simulink model "Lightning_McSeas_VCU"  (R2021b)
settings: Solver=FixedStepDiscrete  StartTime=0.0  StopTime=10.0  FixedStep=0.01  RelTol=1e-3  EnableMultiTasking=on
PreLoadFcn:
  | try, model_open; catch, disp('Error occurred while executing model pre-load callback: model_open.m'); disp('Please assure that the MATLAB working directory is set to the model directory before opening.'); end
InitFcn:
  | try, model_open; catch, end
undefined symbols (not defined in the file): dataName, enumName, enumValue, GCM, raptor_get_safe_string
libraries: Raptor_lib x67, simulink x8
(part 3 of 3)

== system Lightning_McSeas_VCU/Foreground/CAN/RC Rx/Battery Switch/If statement for on off switch/If Action Subsystem ==
  Xa : Inport
  Action Port : ActionPort  ActionPortLabel=if(u1 > 1400)
  Out1 : Outport
  wires:
  Xa/1 -> Out1/1

== system Lightning_McSeas_VCU/Foreground/CAN/RC Rx/Battery Switch/If statement for on off switch/If Action Subsystem1 ==
  Xb : Inport
  Action Port : ActionPort  ActionPortLabel=else
  Out1 : Outport
  wires:
  Xb/1 -> Out1/1

== system Lightning_McSeas_VCU/Foreground/CAN/RC Rx/MCU/If statement for on off switch1/If Action Subsystem ==
  Xa : Inport
  Action Port : ActionPort  ActionPortLabel=if(250 >u1 > 1400)
  Out1 : Outport
  wires:
  Xa/1 -> Out1/1

== system Lightning_McSeas_VCU/Foreground/CAN/RC Rx/MCU/If statement for on off switch1/If Action Subsystem1 ==
  Xb : Inport
  Action Port : ActionPort  ActionPortLabel=else
  Out1 : Outport
  wires:
  Xb/1 -> Out1/1

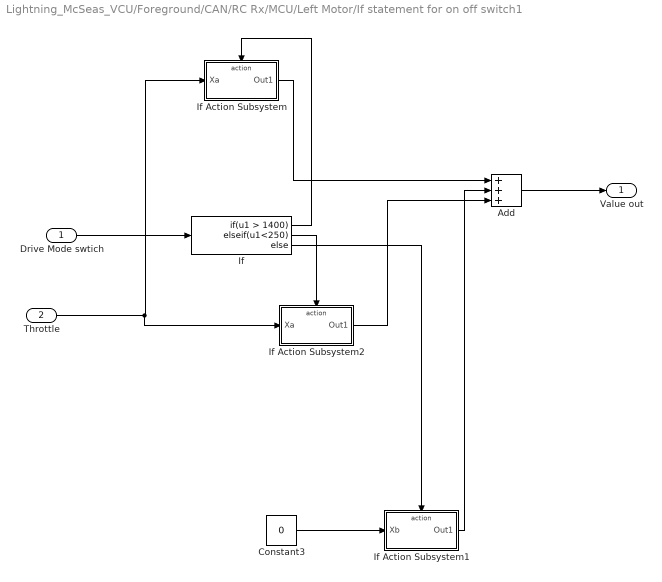
== system Lightning_McSeas_VCU/Foreground/CAN/RC Rx/MCU/Left Motor/If statement for on off switch1 ==
  Drive Mode swtich : Inport
  Throttle : Inport  Port=2
  Add : Sum  Inputs=+++
  Constant3 : Constant  Value=0
  If : If  IfExpression=u1 > 1400  ElseIfExpressions=u1<250
  If Action Subsystem : Subsystem  TreatAsAtomicUnit=on
  If Action Subsystem1 : Subsystem  TreatAsAtomicUnit=on
  If Action Subsystem2 : Subsystem  TreatAsAtomicUnit=on
  Value out : Outport
  wires:
  If Action Subsystem1/1(Out1) -> Add/2
  Add/1 -> Value out/1
  If/1 -> If Action Subsystem/Action
  Constant3/1 -> If Action Subsystem1/1(Xb)
  If Action Subsystem/1(Out1) -> Add/1
  If/3 -> If Action Subsystem1/Action
  Drive Mode swtich/1 -> If/1
  If/2 -> If Action Subsystem2/Action
  If Action Subsystem2/1(Out1) -> Add/3
  Throttle/1 -> If Action Subsystem2/1(Xa), If Action Subsystem/1(Xa)

== system Lightning_McSeas_VCU/Foreground/CAN/RC Rx/MCU/Right Motor/If statement for on off switch1 ==
  Drive Mode swtich : Inport
  Throttle : Inport  Port=2
  Add : Sum  Inputs=+++
  Constant3 : Constant  Value=0
  If : If  IfExpression=u1 > 1400  ElseIfExpressions=u1<250
  If Action Subsystem : Subsystem  TreatAsAtomicUnit=on
  If Action Subsystem1 : Subsystem  TreatAsAtomicUnit=on
  If Action Subsystem2 : Subsystem  TreatAsAtomicUnit=on
  Value out : Outport
  wires:
  If Action Subsystem1/1(Out1) -> Add/2
  Add/1 -> Value out/1
  If/1 -> If Action Subsystem/Action
  Constant3/1 -> If Action Subsystem1/1(Xb)
  If Action Subsystem/1(Out1) -> Add/1
  If/3 -> If Action Subsystem1/Action
  Drive Mode swtich/1 -> If/1
  If/2 -> If Action Subsystem2/Action
  If Action Subsystem2/1(Out1) -> Add/3
  Throttle/1 -> If Action Subsystem2/1(Xa), If Action Subsystem/1(Xa)

== system Lightning_McSeas_VCU/Foreground/CAN/RC Rx/MCU/Left Motor/If statement for on off switch1/If Action Subsystem ==
  Xa : Inport
  Action Port : ActionPort  ActionPortLabel=if(u1 > 1400)
  Out1 : Outport
  wires:
  Xa/1 -> Out1/1

== system Lightning_McSeas_VCU/Foreground/CAN/RC Rx/MCU/Left Motor/If statement for on off switch1/If Action Subsystem1 ==
  Xb : Inport
  Action Port : ActionPort  ActionPortLabel=else
  Out1 : Outport
  wires:
  Xb/1 -> Out1/1

== system Lightning_McSeas_VCU/Foreground/CAN/RC Rx/MCU/Left Motor/If statement for on off switch1/If Action Subsystem2 ==
  Xa : Inport
  Action Port : ActionPort  ActionPortLabel=elseif(u1<250)
  Constant : Constant  Value=-1
  Product : Product
  Out1 : Outport
  wires:
  Xa/1 -> Product/1
  Product/1 -> Out1/1
  Constant/1 -> Product/2

== system Lightning_McSeas_VCU/Foreground/CAN/RC Rx/MCU/Right Motor/If statement for on off switch1/If Action Subsystem ==
  Xa : Inport
  Action Port : ActionPort  ActionPortLabel=if(u1 > 1400)
  Out1 : Outport
  wires:
  Xa/1 -> Out1/1

== system Lightning_McSeas_VCU/Foreground/CAN/RC Rx/MCU/Right Motor/If statement for on off switch1/If Action Subsystem1 ==
  Xb : Inport
  Action Port : ActionPort  ActionPortLabel=else
  Out1 : Outport
  wires:
  Xb/1 -> Out1/1

== system Lightning_McSeas_VCU/Foreground/CAN/RC Rx/MCU/Right Motor/If statement for on off switch1/If Action Subsystem2 ==
  Xa : Inport
  Action Port : ActionPort  ActionPortLabel=elseif(u1<250)
  Constant : Constant  Value=-1
  Product : Product
  Out1 : Outport
  wires:
  Xa/1 -> Product/1
  Product/1 -> Out1/1
  Constant/1 -> Product/2
